simulink model "testesimulink2014"  (R2014b)
settings: Solver=ode45  SolverMode=SingleTasking  StartTime=0.0  StopTime=10.0  RelTol=1e-3
values from neighbouring files (symbols this model uses):
  A = [0 1; -3 -5]    [exemplo.m]    (also in lista_1_func.m = [0 1; 0 -b/m]; lista_2_func.m = [0 1 0; 0 0 1; -6 -11 -6]; lista_4_func.m = [0 1;-w0^2 1]; lista_4_funcv2.m = [0 1;-w0^2 1])
  B = [0;1]    [exemplo.m]    (also in lista_1_func.m = [0;1/m]; lista_2_func.m = [0;0;6]; lista_4_func.m; lista_4_funcv2.m)
  C = [1 0]    [exemplo.m]    (also in lista_1_func.m = [0 1]; lista_2_func.m = [1 0 0]; lista_4_func.m; lista_4_funcv2.m)
  D = 0    [exemplo.m]    (also in lista_1_func.m; lista_2_func.m; lista_4_func.m; lista_4_funcv2.m)
  K = K_Ke(1:end-1)    [designController.m]    (also in lista_4_func.m = acker(A,B,polos); lista_6_v2.m; testesimulinkcode.m = [-775.7143 -20.6429 0.4000])
  L = acker(Ao',Co',polos)'    [designObserver.m]    (also in lista_5_func.m; testesimulinkcode.m = [203;31582;1128200])
settings Model: CovMetricSettings=dwe  CovHtmlReporting=off  covSaveCumulativeToWorkspaceVar=off  CovSaveSingleToWorkspaceVar=off  CovExternalEMLEnable=on  CovSFcnEnable=on  Creator=valdir  LastModifiedBy=valdir
settings DataIOCC: LimitDataPoints=off  SaveFormat=StructureWithTime
settings DebuggingCC: SolverPrmCheckMsg=none  FrameProcessingCompatibilityMsg=error  SFUnexpectedBacktrackingDiag=error  SFNoUnconditionalDefaultTransitionDiag=error
settings HardwareCC: ProdBitPerPointer=64  ProdLargestAtomicFloat=Float  ProdIntDivRoundTo=Zero  ProdEndianess=LittleEndian  ProdHWDeviceType=Specified
settings ModelReferenceCC: PropagateSignalLabelsOutOfModel=on
settings SFSimCC: SimUseLocalCustomCode=on
settings RTWCC: RTWUseLocalCustomCode=on
settings GRTTargetCC: TargetLangStandard=C99 (ISO)  GeneratePreprocessorConditionals=Use local settings

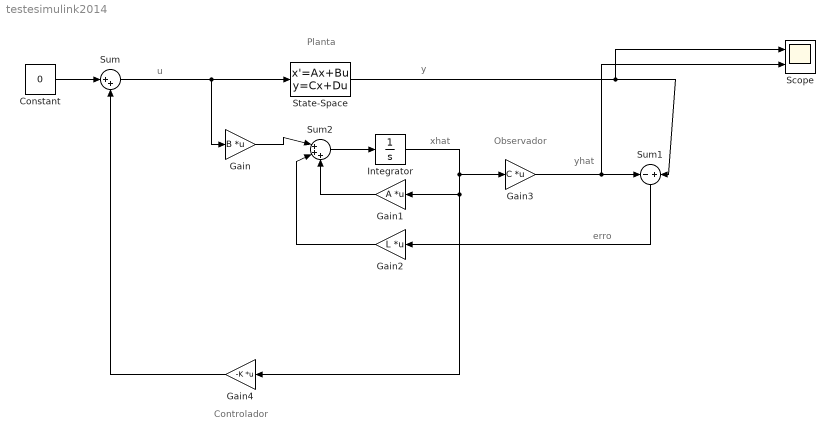
== system testesimulink2014 ==
  note: yhat
  note: y
  note: u
  note: Planta
  note: Observador
  note: Controlador
  note: erro
  note: xhat
  Constant : Constant  Value=0
  Gain : Gain  Gain=B  Multiplication=Matrix(K*u)
  Gain1 : Gain  Gain=A  Multiplication=Matrix(K*u)
  Gain2 : Gain  Gain=L  Multiplication=Matrix(K*u)
  Gain3 : Gain  Gain=C  Multiplication=Matrix(K*u)
  Gain4 : Gain  Gain=-K  Multiplication=Matrix(K*u)
  Integrator : Integrator
  Scope : Scope  NumInputPorts=2
      settings: TimeRange=auto  MaxDataPoints=5000  SaveToWorkspace=off  SaveName=ScopeData  YMin=-1.00000~-5  YMax=1.00000~5  SampleTime=-1
  State-Space : StateSpace  A=A  B=B  C=C  D=D  X0=0
  Sum : Sum  Inputs=|++
  Sum1 : Sum  Inputs=-+
  Sum2 : Sum  Inputs=|+++
  wires:
  Gain4/1 -> Sum/2
  Sum/1 -> Gain/1, State-Space/1
  Gain/1 -> Sum2/1
  Sum2/1 -> Integrator/1
  Integrator/1 -> Gain3/1, Gain4/1, Gain1/1
  Gain1/1 -> Sum2/3
  Gain2/1 -> Sum2/2
  Sum1/1 -> Gain2/1
  State-Space/1 -> Scope/1, Sum1/2
  Constant/1 -> Sum/1
  Gain3/1 -> Scope/2, Sum1/1
